simulink model "HSat_orbit_merged_maria"  (R2023b)
settings: Solver=FixedStepAuto  StartTime=0  StopTime=86400*900  MaxStep=3600  RelTol=1e-3  EnableMultiTasking=on
values from neighbouring files (symbols this model uses):
  alpha_acc = sqrt(0.7)    [HSat_op_setup_merged_maria.m]    (also in init_orbit_analysis_with_drag_loss.m)
  ext_ENV_G = 6.674e-11    [HSat_op_setup.m]    (also in HSat_op_setup_merged_maria.m)
  ext_ENV_muEarth = 3.986005e14    (= 398600500000000)    [GEO_insertion_setup.m]    (also in HSat_op_setup.m; HSat_op_setup_merged_maria.m; init_orbit_analysis_with_drag_loss.m)
  ext_ENV_Re = 6.37813700*10^6    (= 6378137)    [HSat_op_setup.m]    (also in HSat_op_setup_merged_maria.m)
  ext_EOR_atmosphere_end = 1000e3    (= 1000000)    [HSat_op_setup.m]    (also in HSat_op_setup_merged_maria.m)
  ext_EOR_perigeeraise_end = 600e3    (= 600000)    [HSat_op_setup.m]    (also in HSat_op_setup_merged_maria.m)
  ext_Main_initDate_IC_T = sim_start    [HSat_op_setup.m]    (also in HSat_op_setup_merged_maria.m)
  ext_SC_activecorr_COE_ECI = [1, 1, 1, 0, 0, 0, 0, 0 ]    [HSat_op_setup.m]    (also in HSat_op_setup_merged_maria.m)
  ext_SC_balanced_COE_ECI = [ .500    0.70    1.100 1 1]    [HSat_op_setup.m]    (also in HSat_op_setup_merged_maria.m = [ 0.10 2.10 1.40    1.0000    1.0000]; launch_settings.m)
  ext_SC_cutofferror_COE_ECI = [150e3, .01, 0.1*pi/180, .1*pi/180,.1*pi/180, 0, 0, 0]    [HSat_op_setup.m]    (also in HSat_op_setup_merged_maria.m)
  ext_SC_init_COE_ECI = [a0,ecc0,i0,an0,ap0,tran0,eccan0,ma0]    [HSat_op_setup.m]    (also in HSat_op_setup_merged_maria.m)
  ext_SC_target_COE_ECI = [a1,ecc1,i1,an1,ap1,tran1,eccan1,ma1]    [HSat_op_setup.m]    (also in HSat_op_setup_merged_maria.m)
  ext_SC_target_lambda = 67*pi/180    (= 1.16937059884)    [HSat_op_setup.m]    (also in HSat_op_setup_merged_maria.m)
  flip_timer = 2*60*60    (= 7200)    [HSat_op_setup_merged_maria.m]
  P_solar = 4.56e-6    (= 4.56e-06)    [HSat_op_setup_merged_maria.m]    (also in init_orbit_analysis_with_drag_loss.m)
  sim_SC_init_CoG_EOR_dry = [-0.00448 0.00106 0.46931]    [HSat_op_setup.m]    (also in HSat_op_setup_merged_maria.m)
  sim_SC_init_CoG_propellant = [0 0 0.24758]    [HSat_op_setup.m]    (also in HSat_op_setup_merged_maria.m)
  sim_SC_init_dry_mass = sim_SC_init_wet_mass-sim_SC_init_propellant_mass    (= 727)    [HSat_op_setup.m]    (also in HSat_op_setup_merged_maria.m = 813.7)
  sim_SC_init_MoI_EOR_wet = [ ... (first row only)    [HSat_op_setup.m]    (also in HSat_op_setup_merged_maria.m; init_orbit_analysis_with_drag_loss.m)
  sim_SC_init_wet_mass = 750    [HSat_op_setup.m]    (also in HSat_op_setup_merged_maria.m)
  sim_thrust_force = [ ... (first row only)    [HSat_op_setup.m]    (also in HSat_op_setup_merged_maria.m)
  sim_thrust_massflow = [ ... (first row only)    [HSat_op_setup.m]    (also in HSat_op_setup_merged_maria.m)
  sim_thrust_vector = [ ... (first row only)    [HSat_op_setup.m]    (also in HSat_op_setup_merged_maria.m)
  sim_thruster_position = [ ... (first row only)    [HSat_op_setup.m]    (also in HSat_op_setup_merged_maria.m)
  sim_ts_save = 60    [HSat_op_setup.m]    (also in HSat_op_setup_merged_maria.m)
  sun_pointing_SA = 0    [HSat_op_setup_merged_maria.m]    (also in init_orbit_analysis_with_drag_loss.m)
  third_body_jupiter = 1    [HSat_op_setup.m]    (also in HSat_op_setup_merged_maria.m)
  third_body_moon = 1    [HSat_op_setup.m]    (also in HSat_op_setup_merged_maria.m)
  third_body_sun = 1    [HSat_op_setup.m]    (also in HSat_op_setup_merged_maria.m)
libraries: aerolibutil x59, simulink x18, matrix_library x16, Toolbox x10, sharedtransform x9, sharedutil x5, aerolibatmos2 x1, simulink_extras x1
(part 3 of 8)

== system HSat_orbit_merged_maria/Subsystem1/Dynamics/Subsystem/3 body perturbation legendre polynomial/Subsystem3 ==
  sat : Inport
  3 body : Inport  Port=2
  mass : Inport  Port=3
  Legendre deg : Inport  Port=4
  Constant : Constant  Value=6.6743e-11
  Divide : Product  Inputs=/*
  Divide1 : Product  Inputs=*/
  Dot Product : DotProduct  OutDataTypeStr=Inherit: Inherit via internal rule
  Dot Product1 : DotProduct  OutDataTypeStr=Inherit: Inherit via internal rule
  Dot Product2 : DotProduct  OutDataTypeStr=Inherit: Inherit via internal rule
  MATLAB Function : MATLAB Function  TreatAsAtomicUnit=on
  Product{,1..3} (4 alike) : Product
  Sqrt : Sqrt
  Sqrt1 : Sqrt
  Subtract : Sum  Inputs=-+
  Subtract1 : Sum  Inputs=+-
  cos angle : Subsystem
  Out1 : Outport
  wires:
  sat/1 -> cos angle/1(sat), Subtract/2, Subtract1/2, Dot Product2/2, Dot Product2/1  "r_sat"
  3 body/1 -> Dot Product1/1, Dot Product/2, Dot Product/1, Dot Product1/2, Subtract1/1, cos angle/2(3 body)  "r_3body"
  cos angle/1(cos angle) -> MATLAB Function/1(costheta)
  Legendre deg/1 -> MATLAB Function/2(degree)
  Divide/1 -> MATLAB Function/3(h)
  mass/1 -> Product/2
  Constant/1 -> Product/1
  Product/1 -> Divide1/1  "mu_3body"
  Divide1/1 -> Product1/1
  Product1/1 -> Out1/1
  MATLAB Function/1(beta) -> Product2/1
  Subtract1/1 -> Product2/2  "r_sat3body"
  Product2/1 -> Subtract/1
  Subtract/1 -> Product1/2
  Dot Product/1 -> Product3/1
  Product3/1 -> Divide1/2
  Dot Product1/1 -> Sqrt/1
  Sqrt/1 -> Divide/1, Product3/2  "| r_3body |"
  Dot Product2/1 -> Sqrt1/1
  Sqrt1/1 -> Divide/2  "| r_sat |"

== system HSat_orbit_merged_maria/Subsystem1/Dynamics/disturbing torques/Atmospheric model/pos_eci to lla ==
  pos_ECI : Inport
  qECI2ECEF : Inport  Port=2
  ECEF Position to LLA : ECEF2LLA
  Mux : Mux  Inputs=2
  Quaternion Rotation : aerolibutil/Quaternion Rotation
  Out1 : Outport
  wires:
  pos_ECI/1 -> Quaternion Rotation/2
  qECI2ECEF/1 -> Quaternion Rotation/1
  Quaternion Rotation/1 -> ECEF Position to LLA/1
  ECEF Position to LLA/1 -> Mux/1
  ECEF Position to LLA/2 -> Mux/2
  Mux/1 -> Out1/1

== system HSat_orbit_merged_maria/Subsystem1/Dynamics/disturbing torques/Disturbing torques/ECI to SCB ==
  qECI2scb : Inport
  N_gg_eci : Inport  Port=2
  L_gg_eci : Inport  Port=3
  L_aero_eci : Inport  Port=4
  L_srp_eci : Inport  Port=5
  N_total_ECI : Inport  Port=6
  L_total_ECI : Inport  Port=7
  Quaternion Rotation{,1..7} (8 alike) : aerolibutil/Quaternion Rotation
  N_gg_scb : Outport
  L_gg_scb : Outport  Port=2
  L_aero_scb : Outport  Port=3
  L_srp_scb : Outport  Port=4
  N_total_scb : Outport  Port=5
  L_total_scb : Outport  Port=6
  wires:
  qECI2scb/1 -> Quaternion Rotation1/1, Quaternion Rotation2/1, Quaternion Rotation3/1, Quaternion Rotation4/1, Quaternion Rotation7/1, Quaternion Rotation6/1, Quaternion Rotation5/1, Quaternion Rotation/1
  N_gg_eci/1 -> Quaternion Rotation/2
  Quaternion Rotation/1 -> N_gg_scb/1
  Quaternion Rotation1/1 -> L_gg_scb/1
  L_gg_eci/1 -> Quaternion Rotation1/2
  Quaternion Rotation2/1 -> ?
  ? -> Quaternion Rotation2/2
  Quaternion Rotation3/1 -> L_aero_scb/1
  L_aero_eci/1 -> Quaternion Rotation3/2
  Quaternion Rotation4/1 -> ?
  ? -> Quaternion Rotation4/2
  Quaternion Rotation5/1 -> L_srp_scb/1
  L_srp_eci/1 -> Quaternion Rotation5/2
  Quaternion Rotation6/1 -> N_total_scb/1
  Quaternion Rotation7/1 -> L_total_scb/1
  L_total_ECI/1 -> Quaternion Rotation7/2
  N_total_ECI/1 -> Quaternion Rotation6/2

== system HSat_orbit_merged_maria/Subsystem1/Dynamics/disturbing torques/Disturbing torques/Gravity gradient torque ==
  qECI2scb : Inport
  pos : Inport  Port=2
  Constant4 : Constant  Value=sim_SC_init_MoI_EOR_wet
  Constant5 : Constant  Value=-5
  Constant6 : Constant  Value=3
  Constant7 : Constant  Value=ext_ENV_muEarth
  Cross Product1 : matrix_library/Cross Product
  Dot Product1 : DotProduct  OutDataTypeStr=Inherit: Inherit via internal rule
  Integrator : Integrator
  Math Function1 : Math  Operator=pow
  Product1 : Product  Inputs=4
  Product2 : Product  Multiplication=Matrix(*)
  Quaternion Inverse : aerolibutil/Quaternion Inverse
  Quaternion Rotation : aerolibutil/Quaternion Rotation
  Quaternion Rotation1 : aerolibutil/Quaternion Rotation
  Sqrt1 : Sqrt
  N_gg_eci : Outport
  L_gg_eci : Outport  Port=2
  wires:
  Constant5/1 -> Math Function1/2
  Sqrt1/1 -> Math Function1/1
  pos/1 -> Quaternion Rotation1/2, Dot Product1/1, Dot Product1/2, Cross Product1/1
  Constant6/1 -> Product1/3
  Math Function1/1 -> Product1/2
  Product1/1 -> Cross Product1/2
  Dot Product1/1 -> Sqrt1/1
  Constant7/1 -> Product1/4
  qECI2scb/1 -> Quaternion Rotation1/1, Quaternion Inverse/1
  Quaternion Inverse/1 -> Quaternion Rotation/1
  Quaternion Rotation/1 -> Product1/1
  Quaternion Rotation1/1 -> Product2/2  "pos_scb"
  Constant4/1 -> Product2/1
  Product2/1 -> Quaternion Rotation/2
  Cross Product1/1 -> Integrator/1, N_gg_eci/1
  Integrator/1 -> L_gg_eci/1

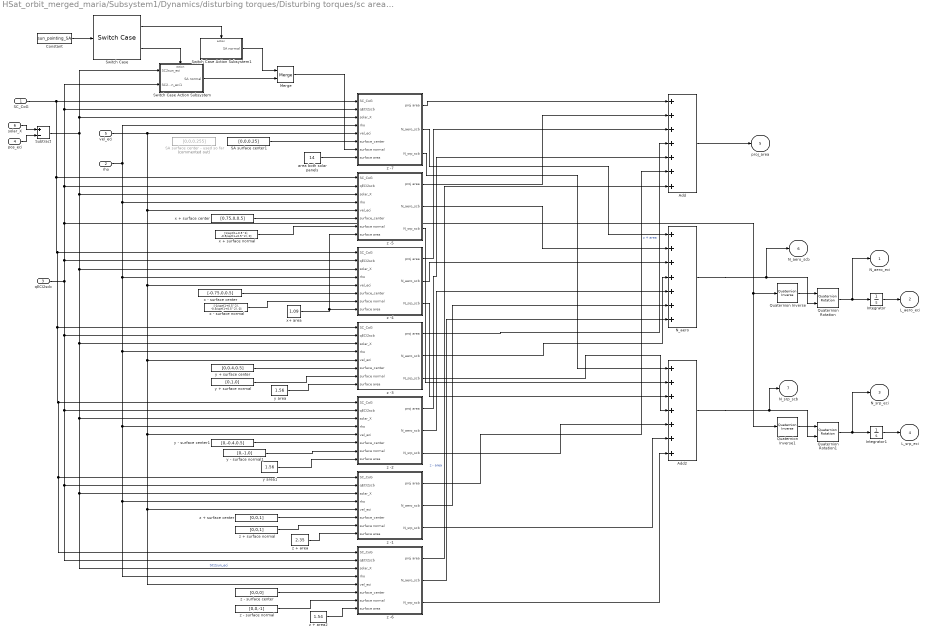
== system HSat_orbit_merged_maria/Subsystem1/Dynamics/disturbing torques/Disturbing torques/sc area projected to v // aero drag torque // srp torque ==
  SC_CoG : Inport
  rho : Inport  Port=2
  qECI2scb : Inport  Port=3
  pos_eci : Inport  Port=4
  vel_eci : Inport  Port=5
  solar_X : Inport  Port=6
  Add : Sum  Inputs=+++++++
  Add2 : Sum  Inputs=+++++++
  Constant : Constant  Value=sun_pointing_SA
  Integrator : Integrator
  Integrator1 : Integrator
  Merge : Merge
  N_aero : Sum  Inputs=+++++++
  Quaternion Inverse : aerolibutil/Quaternion Inverse
  Quaternion Inverse1 : aerolibutil/Quaternion Inverse
  Quaternion Rotation : aerolibutil/Quaternion Rotation
  Quaternion Rotation1 : aerolibutil/Quaternion Rotation
  SA surface center - used so far : Constant  Commented=on  Value=[0,0,0.255]
  SA surface center1 : Constant  Value=[0,0,0.25]
  Subtract : Sum  Inputs=+-
  Switch Case : SwitchCase
  Switch Case Action Subsystem : Subsystem  TreatAsAtomicUnit=on
  Switch Case Action Subsystem1 : Subsystem  TreatAsAtomicUnit=on
  area both solar panels : Constant  Value=14
  x + surface center : Constant  Value=[0.75,0,0.5]
  x + surface normal : Constant  Value=[1/sqrt(1+0.5^2), -0.5/sqrt(1+0.5^2), 0]
  x - surface center : Constant  Value=[-0.75,0,0.5]
  x - surface normal : Constant  Value=[-1/sqrt(1+0.5^2), -0.5/sqrt(1+0.5^2), 0]
  x+ area : Constant  Value=1.09
  y + surface center : Constant  Value=[0,0.4,0.5]
  y + surface normal : Constant  Value=[0,1,0]
  y - surface center1 : Constant  Value=[0,-0.4,0.5]
  y - surface normal1 : Constant  Value=[0,-1,0]
  y area : Constant  Value=1.56
  y area1 : Constant  Value=1.56
  z + area : Constant  Value=2.35
  z + area2 : Constant  Value=1.54
  z + surface center : Constant  Value=[0,0,1]
  z + surface normal : Constant  Value=[0,0,1]
  z - surface center : Constant  Value=[0,0,0]
  z - surface normal : Constant  Value=[0,0,-1]
  z -1 : Subsystem
  z -2 : Subsystem
  z -3 : Subsystem
  z -4 : Subsystem
  z -5 : Subsystem
  z -6 : Subsystem
  z -7 : Subsystem
  N_aero_eci : Outport
  L_aero_eci : Outport  Port=2
  N_srp_eci : Outport  Port=3
  L_srp_eci : Outport  Port=4
  proj_area : Outport  Port=5
  N_aero_scb : Outport  Port=6
  N_srp_scb : Outport  Port=7
  wires:
  z -1/1(proj area) -> Add/6  "z + area"
  Add/1 -> proj_area/1
  area both solar panels/1 -> z -7/8(surface area)
  Subtract/1 -> Switch Case Action Subsystem/1(SC2sun_eci), z -7/3(solar_X), z -5/3(solar_X), z -4/3(solar_X), z -3/3(solar_X), z -2/3(solar_X), z -6/3(solar_X), z -1/3(solar_X)  "SC2sun_eci"
  z -6/1(proj area) -> Add/7  "z - area"
  z - surface normal/1 -> z -6/7(surface normal)
  z + area2/1 -> z -6/8(surface area)
  z - surface center/1 -> z -6/6(surface_center)
  z + surface normal/1 -> z -1/7(surface normal)
  z + area/1 -> z -1/8(surface area)
  z + surface center/1 -> z -1/6(surface_center)
  y + surface normal/1 -> z -3/7(surface normal)
  y area/1 -> z -3/8(surface area)
  y + surface center/1 -> z -3/6(surface_center)
  y - surface normal1/1 -> z -2/7(surface normal)
  y - surface center1/1 -> z -2/6(surface_center)
  rho/1 -> z -7/4(rho), z -5/4(rho), z -4/4(rho), z -3/4(rho), z -2/4(rho), z -6/4(rho), z -1/4(rho)
  y area1/1 -> z -2/8(surface area)
  z -2/1(proj area) -> Add/5
  vel_eci/1 -> z -5/5(vel_eci), z -4/5(vel_eci), z -3/5(vel_eci), z -2/5(vel_eci), z -6/5(vel_eci), z -1/5(vel_eci), z -7/5(vel_eci)
  z -3/1(proj area) -> Add/4
  x - surface normal/1 -> z -4/7(surface normal)
  x - surface center/1 -> z -4/6(surface_center)
  x+ area/1 -> z -4/8(surface area), z -5/8(surface area)
  x + surface normal/1 -> z -5/7(surface normal)
  x + surface center/1 -> z -5/6(surface_center)
  z -4/1(proj area) -> Add/3
  z -5/1(proj area) -> Add/2
  z -5/2(N_aero_scb) -> N_aero/2
  z -4/2(N_aero_scb) -> N_aero/3
  z -3/2(N_aero_scb) -> N_aero/4
  z -2/2(N_aero_scb) -> N_aero/5
  z -1/2(N_aero_scb) -> N_aero/6
  z -6/2(N_aero_scb) -> N_aero/7
  SA surface center1/1 -> z -7/6(surface_center)
  z -7/1(proj area) -> Add/1
  z -7/2(N_aero_scb) -> N_aero/1
  N_aero/1 -> N_aero_scb/1, Quaternion Rotation/2
  Quaternion Rotation/1 -> N_aero_eci/1, Integrator/1
  Integrator/1 -> L_aero_eci/1
  Quaternion Inverse/1 -> Quaternion Rotation/1
  Add2/1 -> N_srp_scb/1, Quaternion Rotation1/2
  Quaternion Inverse1/1 -> Quaternion Rotation1/1
  Quaternion Rotation1/1 -> N_srp_eci/1, Integrator1/1
  qECI2scb/1 -> z -3/2(qECI2scb), z -2/2(qECI2scb), z -6/2(qECI2scb), z -1/2(qECI2scb), Switch Case Action Subsystem/2(SC2sun_eci1), z -7/2(qECI2scb), z -5/2(qECI2scb), Quaternion Inverse1/1, Quaternion Inverse/1, z -4/2(qECI2scb)
  Integrator1/1 -> L_srp_eci/1
  z -7/3(N_srp_scb) -> Add2/1
  z -5/3(N_srp_scb) -> Add2/2
  z -4/3(N_srp_scb) -> Add2/3
  z -3/3(N_srp_scb) -> Add2/4
  z -2/3(N_srp_scb) -> Add2/5
  z -1/3(N_srp_scb) -> Add2/6
  z -6/3(N_srp_scb) -> Add2/7
  solar_X/1 -> Subtract/1
  pos_eci/1 -> Subtract/2
  Switch Case Action Subsystem/1(SA normal) -> Merge/2
  Switch Case/2 -> Switch Case Action Subsystem/Action
  Switch Case/1 -> Switch Case Action Subsystem1/Action
  Switch Case Action Subsystem1/1(SA normal) -> Merge/1
  Merge/1 -> z -7/7(surface normal)
  Constant/1 -> Switch Case/1
  SC_CoG/1 -> z -6/1(SC_CoG), z -1/1(SC_CoG), z -2/1(SC_CoG), z -3/1(SC_CoG), z -4/1(SC_CoG), z -5/1(SC_CoG), z -7/1(SC_CoG)

== system HSat_orbit_merged_maria/Subsystem1/Guidance/Subsystem1/Subsystem/Subsystem1 ==
  lambdadot_guide : Inport
  Constant1 : Constant  Value=2*pi
  Constant5 : Constant  Value=2*pi*86164
  Constant6 : Constant  Value=ext_ENV_muEarth
  Constant7 : Constant  Value=1/3
  Constant8 : Constant  Value=2*pi
  Divide1 : Product  Inputs=**
  Divide2 : Product  Inputs=*/
  Divide3 : Product  Inputs=*/
  Gain : Gain
  Math Function4 : Math  Operator=square
  Math Function5 : Math  Operator=pow
  Subtract1 : Sum
  a_guide : Outport
  wires:
  Constant6/1 -> Divide1/2
  Divide1/1 -> Math Function5/1
  Constant7/1 -> Math Function5/2
  lambdadot_guide/1 -> Gain/1
  Math Function4/1 -> Divide1/1
  Math Function5/1 -> a_guide/1
  Constant8/1 -> Subtract1/2
  Subtract1/1 -> Divide2/2
  Divide2/1 -> Divide3/1  "T-period"
  Constant5/1 -> Divide2/1
  Constant1/1 -> Divide3/2
  Divide3/1 -> Math Function4/1  "T-period"
  Gain/1 -> Subtract1/1

== system HSat_orbit_merged_maria/Subsystem1/Guidance/Subsystem1/Subsystem/plusminuspi ==
  lambda : Inport
  Constant1 : Constant  Value=2*pi
  Constant2 : Constant  Value=2*pi
  Constant4 : Constant  Value=2*pi
  Constant5 : Constant  Value=pi
  Math Function1 : Math  Operator=mod
  Math Function2 : Math  Operator=mod
  Math Function3 : Math  Operator=mod
  Sum11 : Sum  Inputs=|+-
  Sum12 : Sum  Inputs=|++
  lambdadot_guide : Outport
  wires:
  Sum11/1 -> Math Function1/1
  Sum12/1 -> Math Function3/1
  Math Function3/1 -> Sum11/1
  Constant5/1 -> Sum12/2, Sum11/2
  Constant4/1 -> Math Function3/2
  lambda/1 -> Math Function2/1
  Constant1/1 -> Math Function1/2
  Math Function2/1 -> Sum12/1
  Constant2/1 -> Math Function2/2
  Math Function1/1 -> lambdadot_guide/1

== system HSat_orbit_merged_maria/Subsystem1/Guidance/Subsystem1/perigeerraise/Subsystem2 ==
  COE : Inport
  Bus Selector : BusSelector  OutputSignals=sms,ecc
  Constant : Constant
  Constant1 : Constant  Value=ext_ENV_Re
  Product : Product
  Product1 : Product
  Sum : Sum  Inputs=|-+
  Sum1 : Sum  Inputs=|++
  Sum2 : Sum  Inputs=|+-
  Sum3 : Sum  Inputs=|+-
  Perigee altitude : Outport
  Apogee altitude : Outport  Port=2
  wires:
  Product1/1 -> Sum3/1
  COE/1 -> Bus Selector/1
  Sum1/1 -> Product1/2
  Product/1 -> Sum2/1
  Constant/1 -> Sum1/2, Sum/2
  Sum/1 -> Product/2
  Bus Selector/1 -> Product1/1, Product/1  "<sms>"
  Sum2/1 -> Perigee altitude/1
  Sum3/1 -> Apogee altitude/1
  Constant1/1 -> Sum2/2, Sum3/2
  Bus Selector/2 -> Sum/1, Sum1/1  "<ecc>"

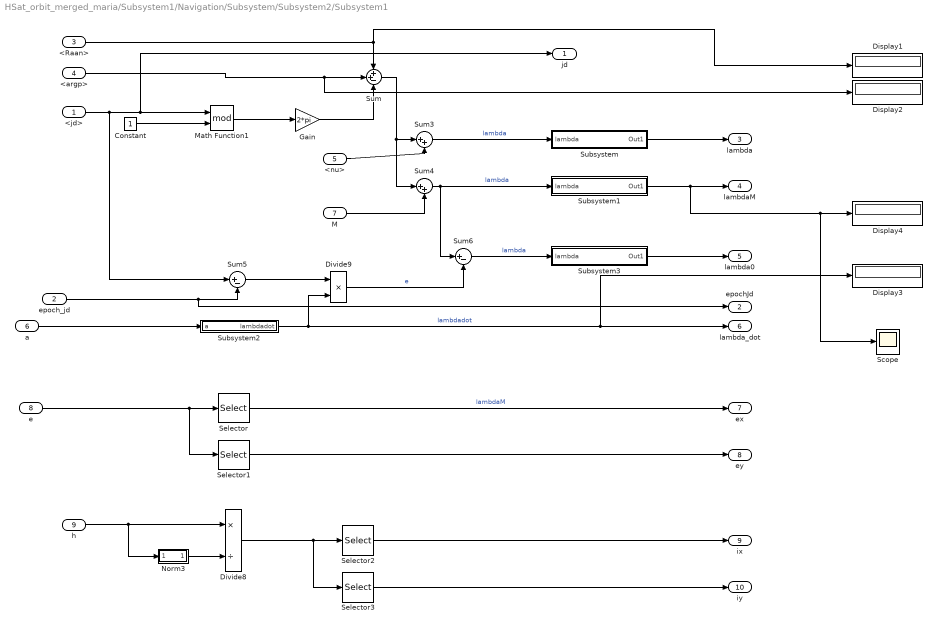
== system HSat_orbit_merged_maria/Subsystem1/Navigation/Subsystem/Subsystem2/Subsystem1 ==
  <jd> : Inport
  epoch_jd : Inport  Port=2
  <Raan> : Inport  Port=3
  <argp> : Inport  Port=4
  <nu> : Inport  Port=5
  a : Inport  Port=6
  M : Inport  Port=7
  e : Inport  Port=8
  h : Inport  Port=9
  Constant : Constant
  Display{1..4} (4 alike) : Display
  Divide8 : Product  Inputs=*/
  Divide9 : Product  Inputs=**
  Gain : Gain  Gain=2*pi
  Math Function1 : Math  Operator=mod
  Norm3 : Subsystem  Tag=||u||
      mask Display: disp('||u||')
  Scope : Scope
  Selector : Selector  InputPortWidth=3  IndexOptions=Index vector (dialog)  Indices=[1]  OutputSizes=1
  Selector1 : Selector  InputPortWidth=3  IndexOptions=Index vector (dialog)  Indices=[2]  OutputSizes=1
  Selector2 : Selector  InputPortWidth=3  IndexOptions=Index vector (dialog)  Indices=[1]  OutputSizes=1
  Selector3 : Selector  InputPortWidth=3  IndexOptions=Index vector (dialog)  Indices=[2]  OutputSizes=1
  Subsystem : Subsystem
  Subsystem1 : Subsystem
  Subsystem2 : Subsystem
  Subsystem3 : Subsystem
  Sum : Sum  Inputs=++-
  Sum3 : Sum  Inputs=|++
  Sum4 : Sum  Inputs=|++
  Sum5 : Sum  Inputs=|+-
  Sum6 : Sum  Inputs=|+-
  jd : Outport
  epochJd : Outport  Port=2
  lambda : Outport  Port=3
  lambdaM : Outport  Port=4
  lambda0 : Outport  Port=5
  lambda_dot : Outport  Port=6
  ex : Outport  Port=7
  ey : Outport  Port=8
  ix : Outport  Port=9
  iy : Outport  Port=10
  wires:
  <Raan>/1 -> Sum/1, Display1/1
  <nu>/1 -> Sum3/2
  Gain/1 -> Sum/3
  Math Function1/1 -> Gain/1
  <jd>/1 -> Sum5/1, Math Function1/1, jd/1
  Constant/1 -> Math Function1/2
  a/1 -> Subsystem2/1(a)
  Sum/1 -> Sum4/1, Sum3/1
  M/1 -> Sum4/2
  epoch_jd/1 -> epochJd/1, Sum5/2
  Sum5/1 -> Divide9/1
  Subsystem2/1(lambdadot) -> Divide9/2, Display3/1, lambda_dot/1  "lambdadot"
  Divide9/1 -> Sum6/2  "e"
  e/1 -> Selector1/1, Selector/1
  Selector1/1 -> ey/1
  Selector/1 -> ex/1  "lambdaM"
  Divide8/1 -> Selector3/1, Selector2/1
  Selector3/1 -> iy/1
  Selector2/1 -> ix/1
  Norm3/1(Out1) -> Divide8/2
  h/1 -> Norm3/1(In1), Divide8/1
  Sum4/1 -> Sum6/1, Subsystem1/1(lambda)  "lambda"
  Sum3/1 -> Subsystem/1(lambda)  "lambda"
  Subsystem/1(Out1) -> lambda/1
  Subsystem1/1(Out1) -> Scope/1, Display4/1, lambdaM/1
  Sum6/1 -> Subsystem3/1(lambda)  "lambda"
  Subsystem3/1(Out1) -> lambda0/1
  <argp>/1 -> Display2/1, Sum/2

== system HSat_orbit_merged_maria/Subsystem1/Navigation/Subsystem/Subsystem2/Subsystem7 ==
  note: ||u||
  r : Inport
  v : Inport  Port=2
  Cross Product : matrix_library/Cross Product
  Norm1 : Subsystem  Tag=||u||
      mask Display: disp('||u||')
  Norm2 : Subsystem  Tag=||u||
      mask Display: disp('||u||')
  Subsystem : Subsystem
  Subsystem1 : Subsystem
  Subsystem2 : Subsystem
  Subsystem3 : Subsystem
  Subsystem4 : Subsystem
  Subsystem5 : Subsystem
  Subsystem6 : Subsystem
  Terminator : Terminator
  a : Outport
  eabs : Outport  Port=2
  i : Outport  Port=3
  Raan : Outport  Port=4
  argp : Outport  Port=5
  nu : Outport  Port=6
  E : Outport  Port=7
  M : Outport  Port=8
  e : Outport  Port=9
  h : Outport  Port=10
  nu igen : Outport  Port=11
  wires:
  Subsystem5/1(nu) -> nu/1
  Subsystem1/3(Raan) -> Raan/1
  Subsystem1/1(N) -> Subsystem4/3(N)  "N"
  Subsystem6/1(a) -> a/1
  Subsystem1/2(N_abs) -> Subsystem4/4(Nabs)  "Nabs"
  Subsystem3/1(e_vec) -> e/1, Subsystem4/1(e), Subsystem5/2(e)  "e"
  Subsystem4/1(argp) -> argp/1
  Norm1/1(Out1) -> Subsystem6/2(vabs), Subsystem3/4(vabs)  "vabs"
  Subsystem2/1(i) -> i/1
  Cross Product/1 -> Subsystem1/1(h), Subsystem2/1(h), h/1  "h"
  v/1 -> Cross Product/2, Subsystem3/3(v), Subsystem/3(v), Norm1/1(In1)
  Subsystem3/2(e_abs) -> eabs/1, Subsystem5/3(eabs), Subsystem4/2(eabs)  "eabs"
  Norm2/1(Out1) -> Subsystem/2(rabs), Subsystem3/2(rabs), Subsystem6/1(rabs), Subsystem5/5(rabs)  "rabs"
  Subsystem5/2(M) -> M/1
  Subsystem5/4(nu igen) -> nu igen/1
  Subsystem5/3(E) -> E/1
  r/1 -> Subsystem/1(r), Norm2/1(In1), Cross Product/1, Subsystem5/4(r), Subsystem3/1(r)
  Subsystem/1(vr) -> Subsystem5/1(vr)
  Subsystem/2(vp) -> Terminator/1

== system HSat_orbit_merged_maria/Subsystem1/control/EORattitude/Subsystem/Subsystem1 ==
  note: the scbp fram is an intemediate frame where:
      | - z is aligned with the resutling thrust,
      | - y is the normalised cross product between the sun vector and z
      | - x completes the orthogonal system
  Flipsign : Inport
  EORthrustSCB : Inport  Port=2
  thrust_slo : Inport  Port=3
  q_slo2eci : Inport  Port=4
  sunv_eci : Inport  Port=5
  Quaternion Inverse : aerolibutil/Quaternion Inverse
  Quaternion Multiplication : aerolibutil/Quaternion Multiplication
  Quaternion Rotation : aerolibutil/Quaternion Rotation
  Subsystem : Subsystem
  q_scb_calc : Subsystem
  qECI2scb : Outport
  wires:
  thrust_slo/1 -> Quaternion Rotation/2
  q_slo2eci/1 -> Quaternion Inverse/1
  sunv_eci/1 -> q_scb_calc/2(sunvECI)
  Quaternion Rotation/1 -> q_scb_calc/1(EORthrustECI)  "vec_eci"
  Quaternion Inverse/1 -> Quaternion Rotation/1
  q_scb_calc/1(qECI2scbp) -> Quaternion Multiplication/1
  Flipsign/1 -> Subsystem/2(Flipsign)
  Subsystem/1(qscbp2scb) -> Quaternion Multiplication/2
  EORthrustSCB/1 -> Subsystem/1(EORthrustSCB)  "thrustscb"
  Quaternion Multiplication/1 -> qECI2scb/1

== system HSat_orbit_merged_maria/Subsystem1/control/EORattitude/Subsystem/Subsystem3 ==
  AmomSCB : Inport
  EORtorqueSCB : Inport  Port=2
  FlipSatellite : Subsystem
  Subsystem : Subsystem
  DoAMOM : Outport
  NoAMOM : Outport  Port=2
  FlipPlusMinus : Outport  Port=3
  wires:
  AmomSCB/1 -> FlipSatellite/1(AmomSCB)
  Subsystem/1(FlipPlusMinus) -> FlipPlusMinus/1
  EORtorqueSCB/1 -> FlipSatellite/2(EORtorqueSCB)
  FlipSatellite/1(FlipSatellite_bool) -> Subsystem/1(FlipNow)
  FlipSatellite/2(DoAMOM) -> DoAMOM/1
  FlipSatellite/3(NoAMOM) -> NoAMOM/1

== system HSat_orbit_merged_maria/Subsystem1/control/EORattitude/Subsystem2/PPU1 ==
  ForceORSCB : Inport
  OR ThrustNo : Inport  Port=2
  TorqueORSCB : Inport  Port=3
  Constant : Constant  Value=[0 0 0 0 0 0 0 0 1 0 0]
  Constant1 : Constant  Value=[0 0 0 0 0 0 0 0 0 0 0]
  Constant2 : Constant  Value=[0 0 0 0 0 0 0 0 0 0 1]
  Demux : Demux  Outputs=3
  Demux1 : Demux  Outputs=3
  Multiport Switch : MultiPortSwitch  SaturateOnIntegerOverflow=off  InputSameDT=off
  Multiport Switch1 : MultiPortSwitch  SaturateOnIntegerOverflow=off  InputSameDT=off
  Multiport Switch2 : MultiPortSwitch  SaturateOnIntegerOverflow=off  InputSameDT=off
  ForceSCB : Outport
  TorqueSCB : Outport  Port=2
  activethrusters : Outport  Port=3
  wires:
  ForceORSCB/1 -> Demux/1
  Demux/1 -> Multiport Switch/2
  Demux/2 -> Multiport Switch/3
  Demux/3 -> Multiport Switch/4
  Multiport Switch/1 -> ForceSCB/1
  Constant1/1 -> Multiport Switch1/3
  Multiport Switch1/1 -> activethrusters/1
  Constant/1 -> Multiport Switch1/2
  Constant2/1 -> Multiport Switch1/4
  Multiport Switch2/1 -> TorqueSCB/1
  TorqueORSCB/1 -> Demux1/1
  Demux1/3 -> Multiport Switch2/4
  Demux1/1 -> Multiport Switch2/2
  OR ThrustNo/1 -> Multiport Switch1/1, Multiport Switch2/1, Multiport Switch/1
  Demux1/2 -> Multiport Switch2/3

== system HSat_orbit_merged_maria/Subsystem1/control/EORattitude/Subsystem2/PPU3 ==
  ForceORSCB : Inport
  OR ThrustNo : Inport  Port=2
  TorqueORSCB : Inport  Port=3
  Constant : Constant  Value=[0 0 0 0 0 0 0 0 0 0 0]
  Constant1 : Constant  Value=[0 0 0 0 0 0 0 0 0 1 0]
  Constant2 : Constant  Value=[0 0 0 0 0 0 0 0 0 0 1]
  Demux : Demux  Outputs=3
  Demux1 : Demux  Outputs=3
  Multiport Switch : MultiPortSwitch  SaturateOnIntegerOverflow=off  InputSameDT=off
  Multiport Switch1 : MultiPortSwitch  SaturateOnIntegerOverflow=off  InputSameDT=off
  Multiport Switch2 : MultiPortSwitch  SaturateOnIntegerOverflow=off  InputSameDT=off
  ForceSCB : Outport
  TorqueSCB : Outport  Port=2
  activethrusters : Outport  Port=3
  wires:
  ForceORSCB/1 -> Demux/1
  Demux/1 -> Multiport Switch/2
  Demux/2 -> Multiport Switch/3
  Demux/3 -> Multiport Switch/4
  Multiport Switch/1 -> ForceSCB/1
  Constant1/1 -> Multiport Switch1/3
  Multiport Switch1/1 -> activethrusters/1
  Constant/1 -> Multiport Switch1/2
  Constant2/1 -> Multiport Switch1/4
  Multiport Switch2/1 -> TorqueSCB/1
  TorqueORSCB/1 -> Demux1/1
  Demux1/3 -> Multiport Switch2/4
  Demux1/1 -> Multiport Switch2/2
  OR ThrustNo/1 -> Multiport Switch1/1, Multiport Switch2/1, Multiport Switch/1
  Demux1/2 -> Multiport Switch2/3

== system HSat_orbit_merged_maria/Subsystem1/control/EORattitude/Subsystem2/PPU_SK ==
  ForceSKSCB : Inport
  SK ThrustNo : Inport  Port=2
  TorqueSKSCB : Inport  Port=3
  Constant : Constant  Value=[1 0 0 0 0 0 0 0 0 0 0]
  Constant1 : Constant  Value=[0 1 0 0 0 0 0 0 0 0 0]
  Constant2 : Constant  Value=[0 0 1 0 0 0 0 0 0 0 0]
  Demux : Demux  Outputs=3
  Demux1 : Demux  Outputs=3
  Multiport Switch : MultiPortSwitch  SaturateOnIntegerOverflow=off  InputSameDT=off
  Multiport Switch1 : MultiPortSwitch  SaturateOnIntegerOverflow=off  InputSameDT=off
  Multiport Switch2 : MultiPortSwitch  SaturateOnIntegerOverflow=off  InputSameDT=off
  ForceSCB : Outport
  TorqueSCB : Outport  Port=2
  activethrusters : Outport  Port=3
  wires:
  ForceSKSCB/1 -> Demux/1
  Demux/1 -> Multiport Switch/2
  Demux/2 -> Multiport Switch/3
  Demux/3 -> Multiport Switch/4
  Multiport Switch/1 -> ForceSCB/1
  Constant1/1 -> Multiport Switch1/3
  Multiport Switch1/1 -> activethrusters/1
  Constant/1 -> Multiport Switch1/2
  Constant2/1 -> Multiport Switch1/4
  Multiport Switch2/1 -> TorqueSCB/1
  TorqueSKSCB/1 -> Demux1/1
  Demux1/3 -> Multiport Switch2/4
  Demux1/1 -> Multiport Switch2/2
  SK ThrustNo/1 -> Multiport Switch1/1, Multiport Switch2/1, Multiport Switch/1
  Demux1/2 -> Multiport Switch2/3

== system HSat_orbit_merged_maria/Subsystem1/control/EORattitude/Subsystem2/thurst and torque for 3 SK thrusters ==
  AllForcesSCB : Inport
  AllTorquesSCB : Inport  Port=2
  ForceSCBOR1 : Selector  NumberOfDimensions=2  InputPortWidth=3  IndexOptions=Index vector (dialog),Index vector (dialog)  Indices=1,[1 2 3]  OutputSizes=1,1
  ForceSCBOR2 : Selector  NumberOfDimensions=2  InputPortWidth=3  IndexOptions=Index vector (dialog),Index vector (dialog)  Indices=2,[1 2 3]  OutputSizes=1,1
  ForceSCBOR3 : Selector  NumberOfDimensions=2  InputPortWidth=3  IndexOptions=Index vector (dialog),Index vector (dialog)  Indices=3,[1 2 3]  OutputSizes=1,1
  Mux : Mux  Inputs=3
  Mux1 : Mux  Inputs=3
  TorqueSCBOR4 : Selector  NumberOfDimensions=2  InputPortWidth=3  IndexOptions=Index vector (dialog),Index vector (dialog)  Indices=1,[1 2 3]  OutputSizes=1,1
  TorqueSCBOR5 : Selector  NumberOfDimensions=2  InputPortWidth=3  IndexOptions=Index vector (dialog),Index vector (dialog)  Indices=2,[1 2 3]  OutputSizes=1,1
  TorqueSCBOR6 : Selector  NumberOfDimensions=2  InputPortWidth=3  IndexOptions=Index vector (dialog),Index vector (dialog)  Indices=3,[1 2 3]  OutputSizes=1,1
  ForceSKSCB : Outport
  TorquesSKSCB : Outport  Port=2
  wires:
  ForceSCBOR3/1 -> Mux/3
  ForceSCBOR2/1 -> Mux/2
  ForceSCBOR1/1 -> Mux/1
  AllForcesSCB/1 -> ForceSCBOR2/1, ForceSCBOR3/1, ForceSCBOR1/1
  Mux/1 -> ForceSKSCB/1
  Mux1/1 -> TorquesSKSCB/1
  TorqueSCBOR4/1 -> Mux1/1
  TorqueSCBOR5/1 -> Mux1/2
  AllTorquesSCB/1 -> TorqueSCBOR5/1, TorqueSCBOR6/1, TorqueSCBOR4/1
  TorqueSCBOR6/1 -> Mux1/3

== system HSat_orbit_merged_maria/Subsystem1/control/EORattitude/Subsystem2/thurst and torque for each OR thruster ==
  AllForcesSCB : Inport
  AllTorquesSCB : Inport  Port=2
  ForceSCBOR1 : Selector  NumberOfDimensions=2  InputPortWidth=3  IndexOptions=Index vector (dialog),Index vector (dialog)  Indices=9,[1 2 3]  OutputSizes=1,1
  ForceSCBOR2 : Selector  NumberOfDimensions=2  InputPortWidth=3  IndexOptions=Index vector (dialog),Index vector (dialog)  Indices=10,[1 2 3]  OutputSizes=1,1
  ForceSCBOR3 : Selector  NumberOfDimensions=2  InputPortWidth=3  IndexOptions=Index vector (dialog),Index vector (dialog)  Indices=11,[1 2 3]  OutputSizes=1,1
  Mux : Mux  Inputs=3
  Mux1 : Mux  Inputs=3
  TorqueSCBOR4 : Selector  NumberOfDimensions=2  InputPortWidth=3  IndexOptions=Index vector (dialog),Index vector (dialog)  Indices=9,[1 2 3]  OutputSizes=1,1
  TorqueSCBOR5 : Selector  NumberOfDimensions=2  InputPortWidth=3  IndexOptions=Index vector (dialog),Index vector (dialog)  Indices=10,[1 2 3]  OutputSizes=1,1
  TorqueSCBOR6 : Selector  NumberOfDimensions=2  InputPortWidth=3  IndexOptions=Index vector (dialog),Index vector (dialog)  Indices=11,[1 2 3]  OutputSizes=1,1
  ForceORSCB : Outport
  TorquesORSCB : Outport  Port=2
  wires:
  ForceSCBOR3/1 -> Mux/3
  ForceSCBOR2/1 -> Mux/2
  ForceSCBOR1/1 -> Mux/1
  AllForcesSCB/1 -> ForceSCBOR2/1, ForceSCBOR3/1, ForceSCBOR1/1
  Mux/1 -> ForceORSCB/1
  Mux1/1 -> TorquesORSCB/1
  TorqueSCBOR4/1 -> Mux1/1
  TorqueSCBOR5/1 -> Mux1/2
  AllTorquesSCB/1 -> TorqueSCBOR5/1, TorqueSCBOR6/1, TorqueSCBOR4/1
  TorqueSCBOR6/1 -> Mux1/3

== system HSat_orbit_merged_maria/Subsystem1/control/EORattitude/Subsystem4/Attitude for OR thrusters ==
  q_eci2slo : Inport
  thrust_vec_slo : Inport  Port=2
  sunvECI : Inport  Port=3
  thrustscb : Inport  Port=4
  Quaternion Inverse : aerolibutil/Quaternion Inverse
  Quaternion Multiplication : aerolibutil/Quaternion Multiplication
  Quaternion Rotation : aerolibutil/Quaternion Rotation
  Subsystem : Subsystem
  q_scb_calc : Subsystem
  q*r : Outport
  wires:
  q_eci2slo/1 -> Quaternion Inverse/1
  Quaternion Multiplication/1 -> q*r/1
  sunvECI/1 -> q_scb_calc/2(sunvECI)
  q_scb_calc/1(qECI2scbp) -> Quaternion Multiplication/1
  thrustscb/1 -> Subsystem/1(EORthrustSCB)
  Quaternion Inverse/1 -> Quaternion Rotation/1  "q_slo2eci"
  Subsystem/1(qscbp2scb) -> Quaternion Multiplication/2
  thrust_vec_slo/1 -> Quaternion Rotation/2
  Quaternion Rotation/1 -> q_scb_calc/1(EORthrustECI)  "vec_eci"

== system HSat_orbit_merged_maria/Subsystem1/control/EORattitude/Subsystem4/Attitude for SK unloading ==
  SKtorqueSCB : Inport
  AmomECI : Inport  Port=2
  sunv_eci : Inport  Port=3
  Direction Cosine Matrix to Quaternions : sharedtransform/Direction Cosine Matrix  to Quaternions  aMode=0  action=None  tolerance=eps(2)
      settings: LibrarySourceBlock=|
      | aerolibtransform2/Direction Cosine Matrix
      | to Quaternions
  Gain : Gain  Gain=-1
  Matrix Concatenate : Concatenate  NumInputs=3  Mode=Multidimensional array
  Quaternion Multiplication : aerolibutil/Quaternion Multiplication
  Reshape1 : Reshape  OutputDimensionality=Row vector (2-D)
  Reshape2 : Reshape  OutputDimensionality=Row vector (2-D)
  Reshape3 : Reshape  OutputDimensionality=Row vector (2-D)
  Subsystem : Subsystem
  VecNormalize : Subsystem
      mask Display: disp('u/||u||')
  VecNormalize1 : Subsystem
      mask Display: disp('u/||u||')
  VecNormalize2 : Subsystem
      mask Display: disp('u/||u||')
  VecNormalize3 : Subsystem
      mask Display: disp('u/||u||')
  Yscb x Zscb : Subsystem  mask(Cross Product){}
      mask help: Calculates the cross product of two 3x1 vectors.
      mask Help:
      | <p>This block calculates the cross product of two 3x1 vectors, ie.</p>
      | 
      | <ul>C(1) = A(2)*B(3) - A(3)*B(2)</ul>
      | <ul>C(2) = A(3)*B(1) - A(1)*B(3)</ul>
      | <ul>C(3) = A(1)*B(2) - A(2)*B(1)</ul>
      | 
      | <p>The block inputs and output contain more than one signal as described below.</p>
      | 
      | <p><H4>Block Vector Input 1 - A</H4>
      | <ul>
      | <li>A(1)</li>
      | <li>A(2)</li>
      | <li>A(3)</li>
      | </ul>
      | </p>
      | 
      | <p><H4>Block Vector Input 2 - B</H4>
      | <ul>
      | <li>B(1)</li>
      | <li>B(2)</li>
      | <li>B(3)</li>
      | </ul>
      | </p>
      | 
      | <p><H4>Block Vector Output - Cross Product (AxB)</H4>
      | <ul>
      | <li>C(1)</li>
      | <li>C(2)</li>
      | <li>C(3)</li>
      | </ul>
      | </p>
      mask Display: disp('Cross\nProduct')
  Zeci x Reci : Subsystem  mask(Cross Product){}
      mask help: Calculates the cross product of two 3x1 vectors.
      mask Help:
      | <p>This block calculates the cross product of two 3x1 vectors, ie.</p>
      | 
      | <ul>C(1) = A(2)*B(3) - A(3)*B(2)</ul>
      | <ul>C(2) = A(3)*B(1) - A(1)*B(3)</ul>
      | <ul>C(3) = A(1)*B(2) - A(2)*B(1)</ul>
      | 
      | <p>The block inputs and output contain more than one signal as described below.</p>
      | 
      | <p><H4>Block Vector Input 1 - A</H4>
      | <ul>
      | <li>A(1)</li>
      | <li>A(2)</li>
      | <li>A(3)</li>
      | </ul>
      | </p>
      | 
      | <p><H4>Block Vector Input 2 - B</H4>
      | <ul>
      | <li>B(1)</li>
      | <li>B(2)</li>
      | <li>B(3)</li>
      | </ul>
      | </p>
      | 
      | <p><H4>Block Vector Output - Cross Product (AxB)</H4>
      | <ul>
      | <li>C(1)</li>
      | <li>C(2)</li>
      | <li>C(3)</li>
      | </ul>
      | </p>
      mask Display: disp('Cross\nProduct')
  q_ECI2scb : Outport
  wires:
  Direction Cosine Matrix to Quaternions/1 -> Quaternion Multiplication/1
  Zeci x Reci/1(c(1) c(2) c(3)) -> VecNormalize3/1(In1)  "Y"
  Reshape2/1 -> Matrix Concatenate/1
  Reshape3/1 -> Matrix Concatenate/3
  sunv_eci/1 -> VecNormalize2/1(In1)
  Reshape1/1 -> Matrix Concatenate/2
  VecNormalize/1(Out1) -> Reshape2/1  "Xscbp"
  VecNormalize2/1(Out1) -> Zeci x Reci/1(a(1) a(2) a(3))
  VecNormalize1/1(Out1) -> Yscb x Zscb/2(b(1) b(2) b(3)), Reshape3/1, Zeci x Reci/2(b(1) b(2) b(3))  "Zscbp"
  AmomECI/1 -> Gain/1
  Yscb x Zscb/1(c(1) c(2) c(3)) -> VecNormalize/1(In1)
  Matrix Concatenate/1 -> Direction Cosine Matrix to Quaternions/1
  VecNormalize3/1(Out1) -> Reshape1/1, Yscb x Zscb/1(a(1) a(2) a(3))  "Yscbp"
  SKtorqueSCB/1 -> Subsystem/1(SKtorqueSCB)  "torque"
  Subsystem/1(qscbp2scb) -> Quaternion Multiplication/2
  Quaternion Multiplication/1 -> q_ECI2scb/1
  Gain/1 -> VecNormalize1/1(In1)

== system HSat_orbit_merged_maria/Subsystem1/control/EORattitude/Subsystem4/Subsystem3 ==
  note: When FlipNow = 1, FlipPlusMinus changes
      | from 0 -> 1 or 1 -> 0.
      | When FlipNow  = 0, FlipPlusMinus keeps the
      | value it has.
  thrustscb : Inport
  AmomECI : Inport  Port=2
  AmomSCB : Inport  Port=3
  EORtorqueSCB : Inport  Port=4
  unloading_ongoing : Inport  Port=5
  Flip satellite based on worst case faior : Subsystem
  FlipSatellite : Subsystem
  Logical Operator1 : Logic  Operator=OR  AllPortsSameDT=off  OutDataTypeStr=boolean
  Manual Switch : ManualSwitch
  Subsystem : Subsystem
  Unit Delay{,1..3} (4 alike) : UnitDelay  SampleTime=-1  HasFrameUpgradeWarning=on
  flip timer and SK trigger : Subsystem
  Flipyaxis : Outport
  DoAMOM : Outport  Port=2
  NoAMOM : Outport  Port=3
  worstRwMom : Outport  Port=4
  SKunload : Outport  Port=5
  idxMinMom : Outport  Port=6
  flip_now : Outport  Port=7
  wires:
  AmomSCB/1 -> Flip satellite based on worst case faior/1(AmomSCB), FlipSatellite/1(AmomSCB)
  Manual Switch/1 -> flip timer and SK trigger/2(flipNow)
  EORtorqueSCB/1 -> FlipSatellite/2(EORtorqueSCB)
  FlipSatellite/1(FlipSatellite_bool) -> Manual Switch/2
  FlipSatellite/2(DoAMOM) -> DoAMOM/1
  FlipSatellite/3(NoAMOM) -> NoAMOM/1
  thrustscb/1 -> Flip satellite based on worst case faior/2(thrustscb)
  Flip satellite based on worst case faior/2(isFlip) -> Manual Switch/1
  Flip satellite based on worst case faior/1(worstRwMom) -> worstRwMom/1, flip timer and SK trigger/6(worstRwMom)
  Subsystem/1(FlipPlusMinus) -> Flipyaxis/1
  flip timer and SK trigger/1(time_integrator) -> Unit Delay/1
  flip timer and SK trigger/2(flip) -> flip_now/1, Subsystem/1(FlipNow)
  flip timer and SK trigger/5(SKunload) -> Logical Operator1/1
  Unit Delay/1 -> flip timer and SK trigger/1(time_int)
  unloading_ongoing/1 -> Logical Operator1/2
  Logical Operator1/1 -> SKunload/1
  Flip satellite based on worst case faior/3(idxMinMom) -> idxMinMom/1
  flip timer and SK trigger/4(counter1) -> Unit Delay1/1
  Unit Delay1/1 -> flip timer and SK trigger/4(counter0)
  flip timer and SK trigger/3(timer1) -> Unit Delay2/1
  Unit Delay2/1 -> flip timer and SK trigger/3(timer0)
  AmomECI/1 -> flip timer and SK trigger/5(AmomECI)
  flip timer and SK trigger/6(time_since_last_flip1) -> Unit Delay3/1
  Unit Delay3/1 -> flip timer and SK trigger/7(time_since_last_flip0)

== system HSat_orbit_merged_maria/Subsystem1/control/EORattitude/Subsystem4/flips around thrust vector ==
  note: Flips SC 180 deg
      | around thrust vector
  thrustscb : Inport
  Constant : Constant  Value=0
  VecNormalize4 : Subsystem
      mask Display: disp('u/||u||')
  Vector Concatenate : Concatenate
  qflipscb : Outport
  wires:
  thrustscb/1 -> VecNormalize4/1(In1)
  Vector Concatenate/1 -> qflipscb/1
  Constant/1 -> Vector Concatenate/1
  VecNormalize4/1(Out1) -> Vector Concatenate/2  "zscbpSCB"

== system HSat_orbit_merged_maria/Subsystem1/control/EORattitude/Subsystem4/use q from thrust calc  ==
  Constant : Constant  Value=[1 0 0 0]
  qflipscb : Outport
  wires:
  Constant/1 -> qflipscb/1

== system HSat_orbit_merged_maria/Subsystem1/control/Subsystem6/Subsystem2/PPU1 ==
  TorqueSKECI : Inport
  WantedTorqueECI : Inport  Port=2
  Constant : Constant  Value=[1 0 0 0 0 0 0 0 0 0 0]
  Constant1 : Constant  Value=[0 0 0 1 0 0 0 0 0 0 0]
  Constant2 : Constant  Value=[0 0 0 0 1 0 0 0 0 0 0]
  Constant3 : Constant  Value=[0 0 0 0 0 0 0 1 0 0 0]
  Demux : Demux  Outputs=8
  Display1 : Display
  Dot Product{,1..3} (4 alike) : DotProduct  OutDataTypeStr=Inherit: Inherit via internal rule
  Multiport Switch : MultiPortSwitch  Inputs=4  SaturateOnIntegerOverflow=off  InputSameDT=off
  Multiport Switch1 : MultiPortSwitch  Inputs=4  SaturateOnIntegerOverflow=off  InputSameDT=off
  Mux : Mux
  Terminator{,1..3} (4 alike) : Terminator
  VecNormalize1 : Subsystem
      mask Display: disp('u/||u||')
  VecNormalize2 : Subsystem
      mask Display: disp('u/||u||')
  VecNormalize3 : Subsystem
      mask Display: disp('u/||u||')
  VecNormalize4 : Subsystem
      mask Display: disp('u/||u||')
  VecNormalize5 : Subsystem
      mask Display: disp('u/||u||')
  VecNormalize6 : Subsystem
      mask Display: disp('u/||u||')
  VecNormalize7 : Subsystem
      mask Display: disp('u/||u||')
  VecNormalize8 : Subsystem
      mask Display: disp('u/||u||')
  find max : Toolbox/vector blocks/find max  SystemSampleTime=-1  VariantActivationTime=update diagram  AllowFlexibleInterface=on  Latency=0  AutoFrameSizeCalculation=off
      settings: SourceProductName=SSC flight toolbox
  torqueSCB : Outport
  activethrusters : Outport  Port=2
  wires:
  TorqueSKECI/1 -> Demux/1
  Demux/2 -> Terminator/1
  Demux/3 -> Terminator1/1
  Demux/6 -> Terminator2/1
  Demux/7 -> Terminator3/1
  Demux/1 -> Multiport Switch/2, VecNormalize2/1(In1)
  Demux/4 -> Multiport Switch/3, VecNormalize4/1(In1)
  Demux/5 -> Multiport Switch/4, VecNormalize6/1(In1)
  Demux/8 -> Multiport Switch/5, VecNormalize8/1(In1)
  WantedTorqueECI/1 -> VecNormalize1/1(In1), VecNormalize3/1(In1), VecNormalize5/1(In1), VecNormalize7/1(In1)
  VecNormalize1/1(Out1) -> Dot Product/1
  VecNormalize2/1(Out1) -> Dot Product/2
  VecNormalize3/1(Out1) -> Dot Product1/1
  VecNormalize4/1(Out1) -> Dot Product1/2
  VecNormalize5/1(Out1) -> Dot Product2/1
  VecNormalize6/1(Out1) -> Dot Product2/2
  VecNormalize7/1(Out1) -> Dot Product3/1
  VecNormalize8/1(Out1) -> Dot Product3/2
  Dot Product/1 -> Mux/1
  Dot Product1/1 -> Mux/2
  Dot Product2/1 -> Mux/3
  Dot Product3/1 -> Mux/4
  Mux/1 -> find max/1
  find max/2 -> Multiport Switch1/1, Multiport Switch/1
  find max/1 -> Display1/1
  Multiport Switch/1 -> torqueSCB/1
  Constant/1 -> Multiport Switch1/2
  Constant1/1 -> Multiport Switch1/3
  Constant2/1 -> Multiport Switch1/4
  Constant3/1 -> Multiport Switch1/5
  Multiport Switch1/1 -> activethrusters/1

== system HSat_orbit_merged_maria/Subsystem1/control/Subsystem6/Subsystem2/PPU1+2 ==
  TorqueSKECI : Inport
  WantedTorqueECI : Inport  Port=2
  Constant : Constant  Value=[1 0 0 0 0 1 0 0 0 0 0]
  Constant1 : Constant  Value=[0 1 0 0 1 0 0 0 0 0 0]
  Constant2 : Constant  Value=[0 0 1 0 0 0 0 1 0 0 0]
  Constant3 : Constant  Value=[0 0 0 1 0 0 1 0 0 0 0]
  Demux : Demux  Outputs=8
  Display1 : Display
  Dot Product{,1..3} (4 alike) : DotProduct  OutDataTypeStr=Inherit: Inherit via internal rule
  Multiport Switch : MultiPortSwitch  Inputs=4  SaturateOnIntegerOverflow=off  InputSameDT=off
  Multiport Switch1 : MultiPortSwitch  Inputs=4  SaturateOnIntegerOverflow=off  InputSameDT=off
  Mux : Mux
  Sum{,1..3} (4 alike) : Sum  Inputs=|++
  VecNormalize1 : Subsystem
      mask Display: disp('u/||u||')
  VecNormalize2 : Subsystem
      mask Display: disp('u/||u||')
  VecNormalize3 : Subsystem
      mask Display: disp('u/||u||')
  VecNormalize4 : Subsystem
      mask Display: disp('u/||u||')
  VecNormalize5 : Subsystem
      mask Display: disp('u/||u||')
  VecNormalize6 : Subsystem
      mask Display: disp('u/||u||')
  VecNormalize7 : Subsystem
      mask Display: disp('u/||u||')
  VecNormalize8 : Subsystem
      mask Display: disp('u/||u||')
  find max : Toolbox/vector blocks/find max  SystemSampleTime=-1  VariantActivationTime=update diagram  AllowFlexibleInterface=on  Latency=0  AutoFrameSizeCalculation=off
      settings: SourceProductName=SSC flight toolbox
  torqueSCB : Outport
  activethrusters : Outport  Port=2
  wires:
  TorqueSKECI/1 -> Demux/1
  Sum1/1 -> Multiport Switch/2, VecNormalize2/1(In1)
  Sum/1 -> Multiport Switch/3, VecNormalize4/1(In1)
  Sum2/1 -> Multiport Switch/4, VecNormalize6/1(In1)
  Sum3/1 -> Multiport Switch/5, VecNormalize8/1(In1)
  WantedTorqueECI/1 -> VecNormalize1/1(In1), VecNormalize3/1(In1), VecNormalize5/1(In1), VecNormalize7/1(In1)
  VecNormalize1/1(Out1) -> Dot Product/1
  VecNormalize2/1(Out1) -> Dot Product/2
  VecNormalize3/1(Out1) -> Dot Product1/1
  VecNormalize4/1(Out1) -> Dot Product1/2
  VecNormalize5/1(Out1) -> Dot Product2/1
  VecNormalize6/1(Out1) -> Dot Product2/2
  VecNormalize7/1(Out1) -> Dot Product3/1
  VecNormalize8/1(Out1) -> Dot Product3/2
  Dot Product/1 -> Mux/1
  Dot Product1/1 -> Mux/2
  Dot Product2/1 -> Mux/3
  Dot Product3/1 -> Mux/4
  Mux/1 -> find max/1
  find max/1 -> Display1/1
  Multiport Switch/1 -> torqueSCB/1
  Demux/4 -> Sum3/1
  Demux/1 -> Sum1/1
  Demux/2 -> Sum/1
  Demux/3 -> Sum2/1
  Demux/6 -> Sum1/2
  Demux/5 -> Sum/2
  Demux/8 -> Sum2/2
  Demux/7 -> Sum3/2
  Constant3/1 -> Multiport Switch1/5
  find max/2 -> Multiport Switch1/1, Multiport Switch/1
  Constant1/1 -> Multiport Switch1/3
  Multiport Switch1/1 -> activethrusters/1
  Constant/1 -> Multiport Switch1/2
  Constant2/1 -> Multiport Switch1/4

== system HSat_orbit_merged_maria/Subsystem1/control/Subsystem6/Subsystem2/PPU2 ==
  TorqueSKECI : Inport
  WantedTorqueECI : Inport  Port=2
  Constant : Constant  Value=[0 1 0 0 0 0 0 0 0 0 0]
  Constant1 : Constant  Value=[0 0 1 0 0 0 0 0 0 0 0]
  Constant2 : Constant  Value=[0 0 0 0 0 1 0 0 0 0 0]
  Constant3 : Constant  Value=[0 0 0 0 0 0 1 0 0 0 0]
  Demux : Demux  Outputs=8
  Display1 : Display
  Dot Product{,1..3} (4 alike) : DotProduct  OutDataTypeStr=Inherit: Inherit via internal rule
  Multiport Switch : MultiPortSwitch  Inputs=4  SaturateOnIntegerOverflow=off  InputSameDT=off
  Multiport Switch1 : MultiPortSwitch  Inputs=4  SaturateOnIntegerOverflow=off  InputSameDT=off
  Mux : Mux
  Terminator{,1..3} (4 alike) : Terminator
  VecNormalize1 : Subsystem
      mask Display: disp('u/||u||')
  VecNormalize2 : Subsystem
      mask Display: disp('u/||u||')
  VecNormalize3 : Subsystem
      mask Display: disp('u/||u||')
  VecNormalize4 : Subsystem
      mask Display: disp('u/||u||')
  VecNormalize5 : Subsystem
      mask Display: disp('u/||u||')
  VecNormalize6 : Subsystem
      mask Display: disp('u/||u||')
  VecNormalize7 : Subsystem
      mask Display: disp('u/||u||')
  VecNormalize8 : Subsystem
      mask Display: disp('u/||u||')
  find max : Toolbox/vector blocks/find max  SystemSampleTime=-1  VariantActivationTime=update diagram  AllowFlexibleInterface=on  Latency=0  AutoFrameSizeCalculation=off
      settings: SourceProductName=SSC flight toolbox
  torqueSCB : Outport
  activethrusters : Outport  Port=2
  wires:
  TorqueSKECI/1 -> Demux/1
  Demux/2 -> VecNormalize2/1(In1), Multiport Switch/2
  Demux/3 -> Multiport Switch/3, VecNormalize4/1(In1)
  Demux/6 -> VecNormalize6/1(In1), Multiport Switch/4
  Demux/7 -> Multiport Switch/5, VecNormalize8/1(In1)
  WantedTorqueECI/1 -> VecNormalize1/1(In1), VecNormalize3/1(In1), VecNormalize5/1(In1), VecNormalize7/1(In1)
  VecNormalize1/1(Out1) -> Dot Product/1
  VecNormalize2/1(Out1) -> Dot Product/2
  VecNormalize3/1(Out1) -> Dot Product1/1
  VecNormalize4/1(Out1) -> Dot Product1/2
  VecNormalize5/1(Out1) -> Dot Product2/1
  VecNormalize6/1(Out1) -> Dot Product2/2
  VecNormalize7/1(Out1) -> Dot Product3/1
  VecNormalize8/1(Out1) -> Dot Product3/2
  Dot Product/1 -> Mux/1
  Dot Product1/1 -> Mux/2
  Dot Product2/1 -> Mux/3
  Dot Product3/1 -> Mux/4
  Mux/1 -> find max/1
  find max/1 -> Display1/1
  Multiport Switch/1 -> torqueSCB/1
  Demux/5 -> Terminator2/1
  Demux/4 -> Terminator1/1
  Demux/1 -> Terminator/1
  Demux/8 -> Terminator3/1
  Multiport Switch1/1 -> activethrusters/1
  Constant/1 -> Multiport Switch1/2
  Constant1/1 -> Multiport Switch1/3
  Constant3/1 -> Multiport Switch1/5
  find max/2 -> Multiport Switch1/1, Multiport Switch/1
  Constant2/1 -> Multiport Switch1/4

== system HSat_orbit_merged_maria/Subsystem1/control/Subsystem6/Subsystem2/Subsystem ==
  AllTorquesSCB : Inport
  q_eci2scb_wanted : Inport  Port=2
  Mux : Mux  Inputs=8
  Quaternion Rotation{,1..7} (8 alike) : aerolibutil/Quaternion Rotation
  TorqueSCBSK1 : Selector  NumberOfDimensions=2  InputPortWidth=3  IndexOptions=Index vector (dialog),Index vector (dialog)  Indices=1,[1 2 3]  OutputSizes=1,1
  TorqueSCBSK2 : Selector  NumberOfDimensions=2  InputPortWidth=3  IndexOptions=Index vector (dialog),Index vector (dialog)  Indices=2,[1 2 3]  OutputSizes=1,1
  TorqueSCBSK3 : Selector  NumberOfDimensions=2  InputPortWidth=3  IndexOptions=Index vector (dialog),Index vector (dialog)  Indices=3,[1 2 3]  OutputSizes=1,1
  TorqueSCBSK4 : Selector  NumberOfDimensions=2  InputPortWidth=3  IndexOptions=Index vector (dialog),Index vector (dialog)  Indices=4,[1 2 3]  OutputSizes=1,1
  TorqueSCBSK5 : Selector  NumberOfDimensions=2  InputPortWidth=3  IndexOptions=Index vector (dialog),Index vector (dialog)  Indices=5,[1 2 3]  OutputSizes=1,1
  TorqueSCBSK6 : Selector  NumberOfDimensions=2  InputPortWidth=3  IndexOptions=Index vector (dialog),Index vector (dialog)  Indices=6,[1 2 3]  OutputSizes=1,1
  TorqueSCBSK7 : Selector  NumberOfDimensions=2  InputPortWidth=3  IndexOptions=Index vector (dialog),Index vector (dialog)  Indices=7,[1 2 3]  OutputSizes=1,1
  TorqueSCBSK8 : Selector  NumberOfDimensions=2  InputPortWidth=3  IndexOptions=Index vector (dialog),Index vector (dialog)  Indices=8,[1 2 3]  OutputSizes=1,1
  TorqueSKECI : Outport
  wires:
  TorqueSCBSK5/1 -> Quaternion Rotation4/2
  Quaternion Rotation3/1 -> Mux/4  "TorqueECISK4"
  Quaternion Rotation6/1 -> Mux/7  "TorqueECISK7"
  Quaternion Rotation4/1 -> Mux/5  "TorqueECISK5"
  TorqueSCBSK3/1 -> Quaternion Rotation2/2
  Quaternion Rotation/1 -> Mux/1  "TorqueECISK1"
  Quaternion Rotation7/1 -> Mux/8  "TorqueECISK8"
  TorqueSCBSK2/1 -> Quaternion Rotation1/2
  Quaternion Rotation2/1 -> Mux/3  "TorqueECISK3"
  TorqueSCBSK4/1 -> Quaternion Rotation3/2
  q_eci2scb_wanted/1 -> Quaternion Rotation7/1, Quaternion Rotation6/1, Quaternion Rotation5/1, Quaternion Rotation4/1, Quaternion Rotation3/1, Quaternion Rotation2/1, Quaternion Rotation1/1, Quaternion Rotation/1
  TorqueSCBSK8/1 -> Quaternion Rotation7/2
  TorqueSCBSK7/1 -> Quaternion Rotation6/2
  TorqueSCBSK1/1 -> Quaternion Rotation/2
  Quaternion Rotation5/1 -> Mux/6  "TorqueECISK6"
  TorqueSCBSK6/1 -> Quaternion Rotation5/2
  AllTorquesSCB/1 -> TorqueSCBSK8/1, TorqueSCBSK7/1, TorqueSCBSK6/1, TorqueSCBSK5/1, TorqueSCBSK4/1, TorqueSCBSK3/1, TorqueSCBSK2/1, TorqueSCBSK1/1
  Quaternion Rotation1/1 -> Mux/2  "TorqueECISK2"
  Mux/1 -> TorqueSKECI/1

== system HSat_orbit_merged_maria/Subsystem1/control/Subsystem6/Subsystem2/Subsystem1 ==
  TorqueSCB : Inport
  WantedTorqueECI : Inport  Port=2
  sunvECI : Inport  Port=3
  Quaternion Multiplication : aerolibutil/Quaternion Multiplication
  Subsystem : Subsystem
  q_scb_calc : Subsystem
  q_eci2scb : Outport
  wires:
  Quaternion Multiplication/1 -> q_eci2scb/1
  sunvECI/1 -> q_scb_calc/2(sunvECI)
  q_scb_calc/1(qECI2scbp) -> Quaternion Multiplication/1
  TorqueSCB/1 -> Subsystem/1(EORthrustSCB)
  Subsystem/1(qscbp2scb) -> Quaternion Multiplication/2
  WantedTorqueECI/1 -> q_scb_calc/1(torqueECI)  "vec_eci"

== system HSat_orbit_merged_maria/Subsystem1/Dynamics/Subsystem/3 body perturbation legendre polynomial/Subsystem1/cos angle ==
  sat : Inport
  3 body : Inport  Port=2
  Divide : Product  Inputs=*//
  Dot Product : DotProduct  OutDataTypeStr=Inherit: Inherit via internal rule
  Dot Product1 : DotProduct  OutDataTypeStr=Inherit: Inherit via internal rule
  Dot Product2 : DotProduct  OutDataTypeStr=Inherit: Inherit via internal rule
  Sqrt : Sqrt
  Sqrt1 : Sqrt
  cos angle : Outport
  wires:
  3 body/1 -> Dot Product1/2, Dot Product1/1, Dot Product/2
  Dot Product1/1 -> Sqrt/1
  sat/1 -> Dot Product/1, Dot Product2/1, Dot Product2/2
  Dot Product2/1 -> Sqrt1/1
  Dot Product/1 -> Divide/1
  Sqrt/1 -> Divide/3
  Sqrt1/1 -> Divide/2
  Divide/1 -> cos angle/1
